simulink model "hw2_q4_redo"  (R2022b)
settings: Solver=ode4  StartTime=0.0  StopTime=10.0  FixedStep=0.001  RelTol=1e-3
settings Model: Creator=gaura  LastModifiedBy=gaura

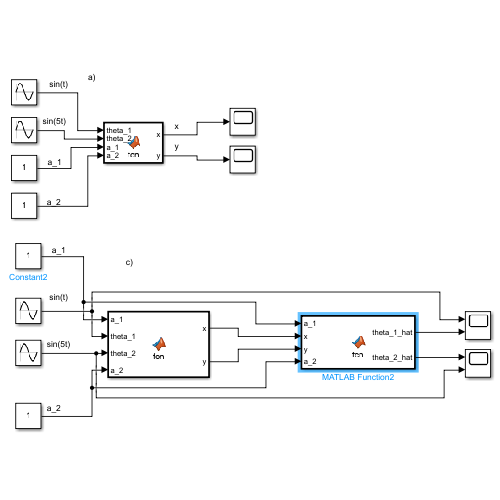
[thumbnail: Simulink's stored preview of the top-level diagram]
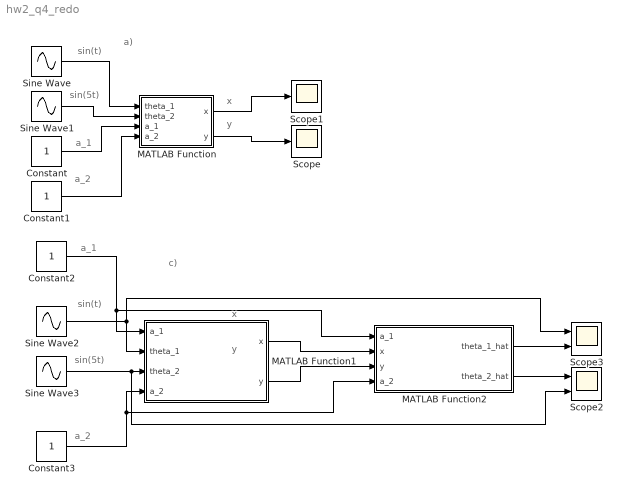
== system hw2_q4_redo ==
  note: c)
  note: a)
  note: sin(t)
  note: sin(5t)
  note: a_2
  note: a_1
  note: y
  note: x
  note: a_2
  note: a_1
  note: sin(t)
  note: y
  note: sin(5t)
  note: x
  Constant{,1..3} (4 alike) : Constant
  MATLAB Function : MATLAB Function  TreatAsAtomicUnit=on
  MATLAB Function1 : MATLAB Function  TreatAsAtomicUnit=on
  MATLAB Function2 : MATLAB Function  TreatAsAtomicUnit=on
  Scope : Scope
  Scope1 : Scope
  Scope2 : Scope  NumInputPorts=2
  Scope3 : Scope  NumInputPorts=2
  Sine Wave : Sin  SampleTime=0
  Sine Wave1 : Sin  Frequency=5  SampleTime=0
  Sine Wave2 : Sin  SampleTime=0
  Sine Wave3 : Sin  Frequency=5  SampleTime=0
  wires:
  MATLAB Function/2(y) -> Scope/1
  Constant/1 -> MATLAB Function/3(a_1)
  Constant1/1 -> MATLAB Function/4(a_2)
  MATLAB Function/1(x) -> Scope1/1
  Sine Wave/1 -> MATLAB Function/1(theta_1)
  Sine Wave1/1 -> MATLAB Function/2(theta_2)
  Sine Wave3/1 -> Scope2/2, MATLAB Function1/3(theta_2)
  Constant3/1 -> MATLAB Function1/4(a_2), MATLAB Function2/4(a_2)
  MATLAB Function1/1(x) -> MATLAB Function2/2(x)
  Constant2/1 -> MATLAB Function1/1(a_1), MATLAB Function2/1(a_1)
  Sine Wave2/1 -> Scope3/1, MATLAB Function1/2(theta_1)
  MATLAB Function1/2(y) -> MATLAB Function2/3(y)
  MATLAB Function2/2(theta_2_hat) -> Scope2/1
  MATLAB Function2/1(theta_1_hat) -> Scope3/2

== matlab function hw2_q4_redo/MATLAB Function1 ==
  data: a_1 input; theta_1 input; x output; theta_2 input; y output; a_2 input
function [x,y] = fcn(a_1, theta_1, theta_2, a_2)

x = a_1*cos(theta_1) + a_2 * cos(theta_1 + theta_2);

y = a_1*sin(theta_1) + a_2 * sin(theta_1 + theta_2);

== matlab function hw2_q4_redo/MATLAB Function ==
  data: theta_1 input; x output; theta_2 input; y output; a_1 input; a_2 input
function [x,y] = fcn(theta_1, theta_2, a_1, a_2)

x = a_1*cos(theta_1) + a_2 * cos(theta_1 + theta_2);

y = a_1*sin(theta_1) + a_2 * sin(theta_1 + theta_2);

== matlab function hw2_q4_redo/MATLAB Function2 ==
  data: a_1 input; x input; y input; theta_1_hat output; a_2 input; theta_2_hat output
function [theta_1_hat, theta_2_hat] = fcn(a_1, x, y, a_2)

D = (x^2 + y^2 - a_1^2 - a_2^2)/(2*a_1*a_2);
s2 = sqrt(1-D.^2);
theta_2_hat = atan2(s2, D);

k1 = a_1 + a_2.*D;
k2 = a_2*s2;
theta_1_hat = atan2(y, x) - atan2(k2, k1);
